simulink model "pSpeedControlSDelay"  (R2014a)
settings: Solver=ode45  StartTime=0.0  StopTime=20.0  RelTol=1e-3
settings Model: Creator=megaman  LastModifiedBy=megaman

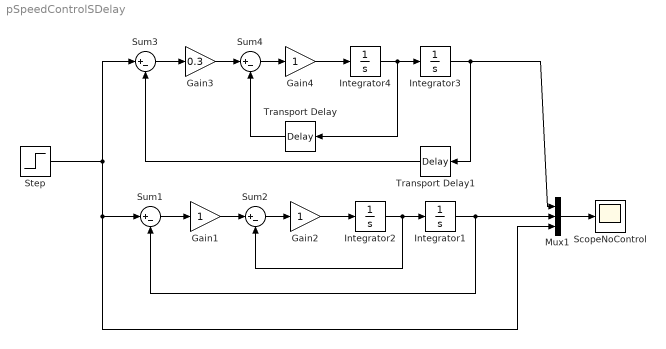
== system pSpeedControlSDelay ==
  Gain1 : Gain
  Gain2 : Gain
  Gain3 : Gain  Gain=0.3
  Gain4 : Gain
  Integrator{1..4} (4 alike) : Integrator
  Mux1 : Mux  Inputs=3
  ScopeNoControl : Scope
      settings: ShowLegends=on
  Step : Step  SampleTime=0
  Sum{1..4} (4 alike) : Sum  Inputs=|+-
  Transport Delay : TransportDelay
  Transport Delay1 : TransportDelay
  wires:
  Integrator1/1 -> Sum1/2, Mux1/2
  Sum1/1 -> Gain1/1
  Step/1 -> Mux1/3, Sum1/1, Sum3/1
  Mux1/1 -> ScopeNoControl/1
  Gain1/1 -> Sum2/1
  Gain2/1 -> Integrator2/1
  Sum2/1 -> Gain2/1
  Integrator2/1 -> Sum2/2, Integrator1/1
  Integrator3/1 -> Transport Delay1/1, Mux1/1
  Sum3/1 -> Gain3/1
  Gain3/1 -> Sum4/1
  Gain4/1 -> Integrator4/1
  Sum4/1 -> Gain4/1
  Integrator4/1 -> Transport Delay/1, Integrator3/1
  Transport Delay/1 -> Sum4/2
  Transport Delay1/1 -> Sum3/2
